simulink model "kal"  (R2020a)
settings: Solver=VariableStepAuto  StartTime=0.0  StopTime=10.0  RelTol=1e-3
undefined symbols (not defined in the file): A, B, C
settings Model: Creator=DEVESH  LastModifiedBy=DEVESH

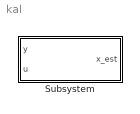
== system kal ==
  Subsystem : Subsystem

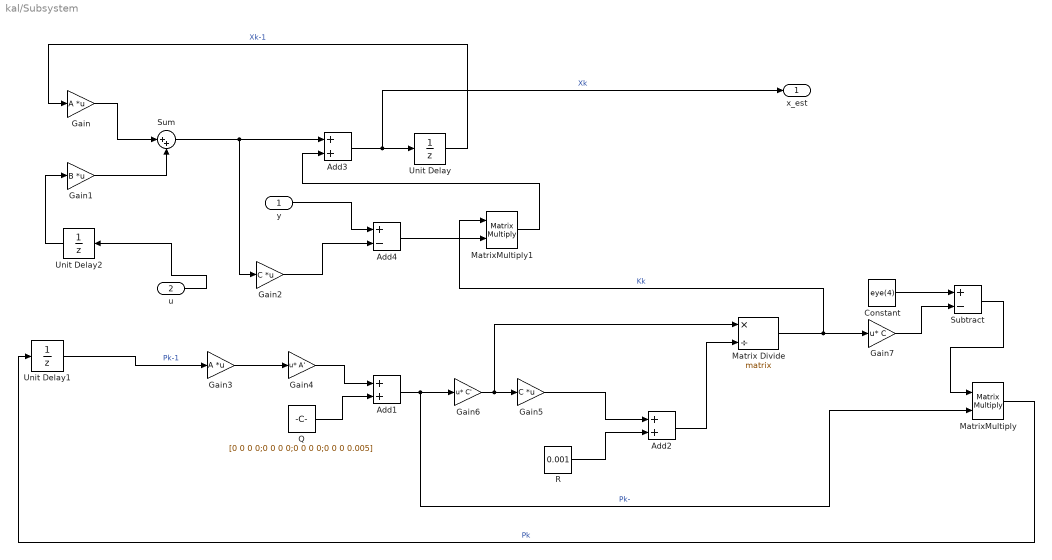
== system kal/Subsystem ==
  y : Inport
  u : Inport  Port=2
  Add1 : Sum
  Add2 : Sum
  Add3 : Sum
  Add4 : Sum  Inputs=+-
  Constant : Constant  Value=eye(4)
  Gain : Gain  Gain=A  Multiplication=Matrix(K*u)
  Gain1 : Gain  Gain=B  Multiplication=Matrix(K*u)
  Gain2 : Gain  Gain=C  Multiplication=Matrix(K*u)
  Gain3 : Gain  Gain=A  Multiplication=Matrix(K*u)
  Gain4 : Gain  Gain=A'  Multiplication=Matrix(u*K)
  Gain5 : Gain  Gain=C  Multiplication=Matrix(K*u)
  Gain6 : Gain  Gain=C'  Multiplication=Matrix(u*K)
  Gain7 : Gain  Gain=C  Multiplication=Matrix(u*K)
  Matrix Divide : Product  Inputs=*/  Multiplication=Matrix(*)
  MatrixMultiply : Product  Multiplication=Matrix(*)
  MatrixMultiply1 : Product  Multiplication=Matrix(*)
  Q : Constant  Value=[0 0 0 0;0 0 0 0;0 0 0 0;0 0 0 0.005]
  R : Constant  Value=0.001
  Subtract : Sum  Inputs=+-
  Sum : Sum  Inputs=|++
  Unit Delay : UnitDelay  InitialCondition=[0;1;0;0]  SampleTime=0.01  HasFrameUpgradeWarning=on
  Unit Delay1 : UnitDelay  SampleTime=0.01  HasFrameUpgradeWarning=on
  Unit Delay2 : UnitDelay  SampleTime=-1  HasFrameUpgradeWarning=on
  x_est : Outport
  wires:
  Add2/1 -> Matrix Divide/2
  Unit Delay/1 -> Gain/1  "Xk-1"
  Gain2/1 -> Add4/2
  Unit Delay1/1 -> Gain3/1  "Pk-1"
  R/1 -> Add2/2
  Gain3/1 -> Gain4/1
  Add1/1 -> MatrixMultiply/2, Gain6/1  "Pk-"
  Matrix Divide/1 -> MatrixMultiply1/1, Gain7/1  "Kk"
  Constant/1 -> Subtract/1
  Gain4/1 -> Add1/1
  Add3/1 -> x_est/1, Unit Delay/1  "Xk"
  MatrixMultiply1/1 -> Add3/2
  Gain5/1 -> Add2/1
  Gain/1 -> Sum/1
  u/1 -> Unit Delay2/1
  Subtract/1 -> MatrixMultiply/1
  Sum/1 -> Gain2/1, Add3/1
  Gain1/1 -> Sum/2
  Gain7/1 -> Subtract/2
  MatrixMultiply/1 -> Unit Delay1/1  "Pk"
  Add4/1 -> MatrixMultiply1/2
  Q/1 -> Add1/2
  y/1 -> Add4/1
  Gain6/1 -> Matrix Divide/1, Gain5/1
  Unit Delay2/1 -> Gain1/1
